simulink model "demodulation"  (R2022b)
settings: Solver=VariableStepAuto  StartTime=0.0  StopTime=1  RelTol=1e-3
libraries: commsynccomp2 x2, dspfdesign x1
settings Model: Creator=Samin  LastModifiedBy=rosie

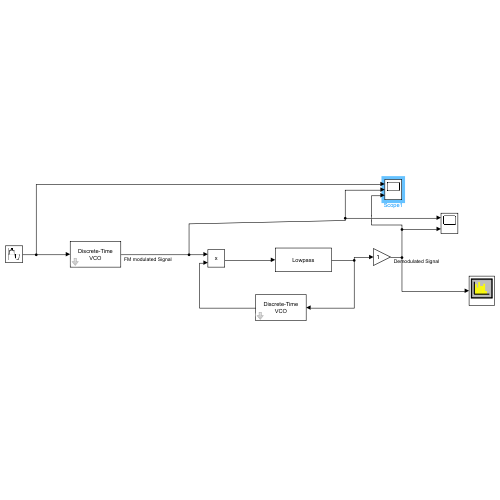
[thumbnail: Simulink's stored preview of the top-level diagram]
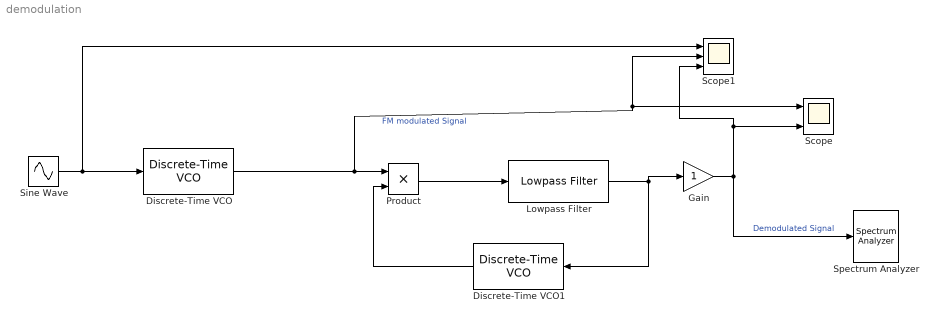
== system demodulation ==
  Discrete-Time VCO : commsynccomp2/Discrete-Time VCO  Ac=1  Fc=10000  Kc=100  Ph=0  ts=1/2e5
  Discrete-Time VCO1 : commsynccomp2/Discrete-Time VCO  Ac=2  Fc=10e3  Kc=100  Ph=0  ts=1/2e5
  Gain : Gain
  Lowpass Filter : dspfdesign/Lowpass Filter  FilterType=FIR  DesignForMinimumOrder=on  FilterOrder=50  PassbandFrequency=2.5e3  StopbandFrequency=3.5e3  PassbandRipple=0.1  StopbandAttenuation=80  InheritSampleRate=on  SampleRate=200e3  SimulateUsing=Interpreted execution  roundingMode=Floor  coeffsDataTypeStr=fixdt(1,16)
  Product : Product  Description=Matrix Multiply
  Scope : Scope  NumInputPorts=2
  Scope1 : Scope  NumInputPorts=3
  Sine Wave : Sin  Frequency=12566.370614  SampleTime=1/2e5
  Spectrum Analyzer : SpectrumAnalyzer
  wires:
  Discrete-Time VCO1/1 -> Product/2
  Sine Wave/1 -> Scope1/1, Discrete-Time VCO/1
  Gain/1 -> Scope/2, Scope1/3, Spectrum Analyzer/1  "Demodulated Signal"
  Lowpass Filter/1 -> Gain/1, Discrete-Time VCO1/1
  Discrete-Time VCO/1 -> Scope/1, Scope1/2, Product/1  "FM modulated Signal"
  Product/1 -> Lowpass Filter/1
